simulink model "Exercise_3"  (R2022a)
settings: Solver=VariableStepAuto  StartTime=0.0  StopTime=10.0  RelTol=1e-3
libraries: simulink x1
settings Model: Creator=Shocky  LastModifiedBy=Shocky

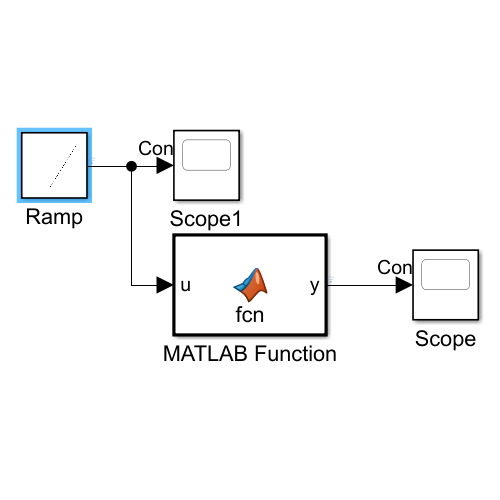
[thumbnail: Simulink's stored preview of the top-level diagram]
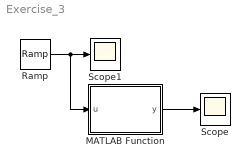
== system Exercise_3 ==
  MATLAB Function : MATLAB Function  TreatAsAtomicUnit=on
  Ramp : simulink/Sources/Ramp  slope=0.5  start=0  InitialOutput=0
  Scope : Scope
  Scope1 : Scope
  wires:
  MATLAB Function/1(y) -> Scope/1
  Ramp/1 -> MATLAB Function/1(u), Scope1/1

== matlab function Exercise_3/MATLAB Function ==
  data: u input; y output
function y = fcn(u)
y=sin(u);
end
